simulink model "SGBMDisparityExample_original"  (R2021a)
settings: Solver=FixedStepDiscrete  StartTime=0.0  StopTime=simT  FixedStep=1  RelTol=1e-3
PreLoadFcn:
  | DL128 = Simulink.Variant('disparityLevels==128');
  | 
  | DLnot128 = Simulink.Variant('disparityLevels ~= 128');
  | 
  | disparityLevels = 64;
  | 
  | imgRowSize = 480;
  | 
  | imgColSize = 640;
  | 
  | P2 = 200; % Smoothness Penalty Large
  | P1 = 15;  % Smoothness Penalty Small
  | 
  | disparityFactor = 16;
  | 
  | uniquenessRatio = 5;
  | 
  | p = imgColSize - 1;
  | q = imgRowSize * imgColSize -1;
  | r = imgColSize - disparityLevels -1;
  | s = (imgRowSize*(imgColSize-disparityLevels))-1;
  | 
  | simT = 800*525
  | 
  | dtGain = 4;
InitFcn:
  | DL128 = Simulink.Variant('disparityLevels==128');
  | 
  | DLnot128 = Simulink.Variant('disparityLevels ~= 128');
  | 
  | img = imread(get_param('SGBMDisparityExample/leftImage','FileName'));
  | 
  | [imgRowSize, imgColSize] = size(img);
  | 
  | P2 = 200; % Smoothness Penalty Large
  | P1 = 15;  % Smoothness Penalty Small
  | 
  | disparityFactor = 16;
  | 
  | uniquenessRatio = str2num(get_param('SGBMDisparityExample/SGBMHDLAlgorithm','UT'));
  | 
  | disparityLevels = str2num(get_param('SGBMDisparityExample/SGBMHDLAlgorithm','DL'));
  | 
  | p = imgColSize - 1;
  | q = imgRowSize * imgColSize -1;
  | r = imgColSize - disparityLevels -1;
  | s = (imgRowSize*(imgColSize-disparityLevels))-1;
  | 
  | if imgRowSize == 720 && imgColSize == 1280
  | simT = 1650*750;
  | elseif imgRowSize == 540 && imgColSize == 960
  | simT = 1050*600;
  | elseif imgRowSize == 480 && imgColSize == 640
  | simT = 800*525;
  | end
  | 
  | if imgRowSize == 720 && imgColSize == 1280
  | dtGain = 2;
  | elseif imgRowSize == 540 && imgColSize == 960
  | dtGain = 2.6;
  | elseif imgRowSize == 480 && imgColSize == 640
  | dtGain = 4;
  | end
libraries: simulink x331, hdlsllib x105, visionhdlutilities x10, visionhdlio x4, visionsources x3
(part 6 of 6)

== system SGBMDisparityExample_original/SGBMHDLAlgorithm/PostProcessing/Interpolation/Division/QuoRem/Last ==
  In1 : Inport
  In2 : Inport  Port=2
  In3 : Inport  Port=3
  Add : Sum  OutDataTypeStr=fixdt(0,13,0)
  Add1 : Sum  Inputs=+-  OutDataTypeStr=fixdt(0,13,0)
  Add2 : Sum  OutDataTypeStr=fixdt(0,13,0)
  Bit Shift : hdlsllib/Logic and Bit Operations/Bit Shift  mode=Shift Left Logical  N=1
  Bitwise Operator : simulink/Logic and Bit Operations/Bitwise Operator  logicop=OR  UseBitMask=on  BitMask=bin2dec('0000')  BitMaskRealWorld=Stored Integer
  Bitwise Operator2 : simulink/Logic and Bit Operations/Bitwise Operator  logicop=OR  UseBitMask=on  BitMask=bin2dec('0001')  BitMaskRealWorld=Stored Integer
  Extract Bits{1..2,5..6} (4 alike) : simulink/Logic and Bit Operations/Extract Bits  bitsToExtract=Range starting with most significant bit  numBits=1  bitIdxRange=[7]  outScalingMode=Treat bit field as an integer
  Extract Bits3 : simulink/Logic and Bit Operations/Extract Bits  bitsToExtract=Upper half  numBits=8  bitIdxRange=[7]  outScalingMode=Treat bit field as an integer
  Extract Bits4 : simulink/Logic and Bit Operations/Extract Bits  bitsToExtract=Lower half  numBits=8  bitIdxRange=[7]  outScalingMode=Treat bit field as an integer
  Logical Operator : Logic  Operator=OR  AllPortsSameDT=off  OutDataTypeStr=boolean
  Switch{,1..4} (5 alike) : Switch  Criteria=u2 ~= 0
  Quo : Outport  VectorParamsAs1DForOutWhenUnconnected=off
  Div : Outport  Port=2  VectorParamsAs1DForOutWhenUnconnected=off
  Rem : Outport  Port=3  VectorParamsAs1DForOutWhenUnconnected=off
  wires:
  Add/1 -> Switch/1
  Bitwise Operator2/1 -> Switch1/3
  Bitwise Operator/1 -> Switch1/1
  Extract Bits2/1 -> Switch1/2
  Add1/1 -> Switch/3
  Extract Bits5/1 -> Switch2/2
  Add2/1 -> Switch2/1
  In1/1 -> Extract Bits1/1, Bit Shift/1
  Bit Shift/1 -> Extract Bits4/1, Extract Bits3/1
  Extract Bits3/1 -> Switch3/3, Add1/1, Add/1
  Extract Bits1/1 -> Switch/2
  Extract Bits4/1 -> Switch4/3, Extract Bits6/1, Bitwise Operator2/1, Bitwise Operator/1
  Switch/1 -> Extract Bits5/1, Add2/1, Extract Bits2/1, Switch2/3
  In2/1 -> Div/1, Add1/2, Add2/2, Add/2
  Switch3/1 -> Rem/1
  Switch4/1 -> Quo/1
  Extract Bits6/1 -> Logical Operator/1
  In3/1 -> Logical Operator/2
  Logical Operator/1 -> Switch3/2, Switch4/2
  Switch1/1 -> Switch4/1
  Switch2/1 -> Switch3/1

== system SGBMDisparityExample_original/SGBMHDLAlgorithm/PostProcessing/Interpolation/Division/QuoRem/Subsystem10 ==
  In1 : Inport
  In2 : Inport  Port=2
  In3 : Inport  Port=3
  Add : Sum  OutDataTypeStr=fixdt(0,13,0)
  Add1 : Sum  Inputs=+-  OutDataTypeStr=fixdt(0,13,0)
  Bit Concat2 : hdlsllib/Logic and Bit Operations/Bit Concat  numInputs=2
  Bit Shift : hdlsllib/Logic and Bit Operations/Bit Shift  mode=Shift Left Logical  N=1
  Bitwise Operator : simulink/Logic and Bit Operations/Bitwise Operator  logicop=OR  UseBitMask=on  BitMask=bin2dec('0')  BitMaskRealWorld=Stored Integer
  Bitwise Operator2 : simulink/Logic and Bit Operations/Bitwise Operator  logicop=OR  UseBitMask=on  BitMask=bin2dec('1')  BitMaskRealWorld=Stored Integer
  Extract Bits1 : simulink/Logic and Bit Operations/Extract Bits  bitsToExtract=Range starting with most significant bit  numBits=1  bitIdxRange=[7]  outScalingMode=Treat bit field as an integer
  Extract Bits2 : simulink/Logic and Bit Operations/Extract Bits  bitsToExtract=Range starting with most significant bit  numBits=1  bitIdxRange=[7]  outScalingMode=Treat bit field as an integer
  Extract Bits3 : simulink/Logic and Bit Operations/Extract Bits  bitsToExtract=Upper half  numBits=8  bitIdxRange=[7]  outScalingMode=Treat bit field as an integer
  Extract Bits4 : simulink/Logic and Bit Operations/Extract Bits  bitsToExtract=Lower half  numBits=8  bitIdxRange=[7]  outScalingMode=Treat bit field as an integer
  Extract Bits5 : simulink/Logic and Bit Operations/Extract Bits  bitsToExtract=Range starting with most significant bit  numBits=1  bitIdxRange=[7]  outScalingMode=Treat bit field as an integer
  Logical Operator : Logic  Operator=OR  AllPortsSameDT=off  OutDataTypeStr=boolean
  Switch : Switch  Criteria=u2 ~= 0
  Switch1 : Switch  Criteria=u2 ~= 0
  Switch2 : Switch  Criteria=u2 ~= 0
  Out1 : Outport  VectorParamsAs1DForOutWhenUnconnected=off
  Out2 : Outport  Port=2  VectorParamsAs1DForOutWhenUnconnected=off
  Start : Outport  Port=3  VectorParamsAs1DForOutWhenUnconnected=off
  wires:
  Add/1 -> Switch/1
  Bitwise Operator2/1 -> Switch1/3
  Bitwise Operator/1 -> Switch1/1
  Extract Bits2/1 -> Switch1/2
  Add1/1 -> Switch/3
  In1/1 -> Extract Bits1/1, Bit Shift/1
  Bit Shift/1 -> Extract Bits4/1, Extract Bits3/1, Switch2/3
  Extract Bits1/1 -> Switch/2
  Extract Bits3/1 -> Add1/1, Add/1
  Switch/1 -> Bit Concat2/1, Extract Bits2/1
  Switch1/1 -> Bit Concat2/2
  In2/1 -> Out2/1, Add1/2, Add/2
  Extract Bits4/1 -> Extract Bits5/1, Bitwise Operator2/1, Bitwise Operator/1
  Switch2/1 -> Out1/1
  Bit Concat2/1 -> Switch2/1
  Extract Bits5/1 -> Logical Operator/1
  In3/1 -> Logical Operator/2
  Logical Operator/1 -> Switch2/2, Start/1

== system SGBMDisparityExample_original/SGBMHDLAlgorithm/PostProcessing/Interpolation/Division/QuoRem/Subsystem11 ==
  In1 : Inport
  In2 : Inport  Port=2
  In3 : Inport  Port=3
  Add : Sum  OutDataTypeStr=fixdt(0,13,0)
  Add1 : Sum  Inputs=+-  OutDataTypeStr=fixdt(0,13,0)
  Bit Concat2 : hdlsllib/Logic and Bit Operations/Bit Concat  numInputs=2
  Bit Shift : hdlsllib/Logic and Bit Operations/Bit Shift  mode=Shift Left Logical  N=1
  Bitwise Operator : simulink/Logic and Bit Operations/Bitwise Operator  logicop=OR  UseBitMask=on  BitMask=bin2dec('0')  BitMaskRealWorld=Stored Integer
  Bitwise Operator2 : simulink/Logic and Bit Operations/Bitwise Operator  logicop=OR  UseBitMask=on  BitMask=bin2dec('1')  BitMaskRealWorld=Stored Integer
  Extract Bits1 : simulink/Logic and Bit Operations/Extract Bits  bitsToExtract=Range starting with most significant bit  numBits=1  bitIdxRange=[7]  outScalingMode=Treat bit field as an integer
  Extract Bits2 : simulink/Logic and Bit Operations/Extract Bits  bitsToExtract=Range starting with most significant bit  numBits=1  bitIdxRange=[7]  outScalingMode=Treat bit field as an integer
  Extract Bits3 : simulink/Logic and Bit Operations/Extract Bits  bitsToExtract=Upper half  numBits=8  bitIdxRange=[7]  outScalingMode=Treat bit field as an integer
  Extract Bits4 : simulink/Logic and Bit Operations/Extract Bits  bitsToExtract=Lower half  numBits=8  bitIdxRange=[7]  outScalingMode=Treat bit field as an integer
  Extract Bits5 : simulink/Logic and Bit Operations/Extract Bits  bitsToExtract=Range starting with most significant bit  numBits=1  bitIdxRange=[7]  outScalingMode=Treat bit field as an integer
  Logical Operator : Logic  Operator=OR  AllPortsSameDT=off  OutDataTypeStr=boolean
  Switch : Switch  Criteria=u2 ~= 0
  Switch1 : Switch  Criteria=u2 ~= 0
  Switch2 : Switch  Criteria=u2 ~= 0
  Out1 : Outport  VectorParamsAs1DForOutWhenUnconnected=off
  Out2 : Outport  Port=2  VectorParamsAs1DForOutWhenUnconnected=off
  Start : Outport  Port=3  VectorParamsAs1DForOutWhenUnconnected=off
  wires:
  Add/1 -> Switch/1
  Bitwise Operator2/1 -> Switch1/3
  Bitwise Operator/1 -> Switch1/1
  Extract Bits2/1 -> Switch1/2
  Add1/1 -> Switch/3
  In1/1 -> Extract Bits1/1, Bit Shift/1
  Bit Shift/1 -> Extract Bits4/1, Extract Bits3/1, Switch2/3
  Extract Bits1/1 -> Switch/2
  Extract Bits3/1 -> Add1/1, Add/1
  Switch/1 -> Bit Concat2/1, Extract Bits2/1
  Switch1/1 -> Bit Concat2/2
  In2/1 -> Out2/1, Add1/2, Add/2
  Extract Bits4/1 -> Extract Bits5/1, Bitwise Operator2/1, Bitwise Operator/1
  Switch2/1 -> Out1/1
  Bit Concat2/1 -> Switch2/1
  Extract Bits5/1 -> Logical Operator/1
  In3/1 -> Logical Operator/2
  Logical Operator/1 -> Switch2/2, Start/1

== system SGBMDisparityExample_original/SGBMHDLAlgorithm/PostProcessing/Interpolation/Division/QuoRem/Subsystem12 ==
  In1 : Inport
  In2 : Inport  Port=2
  In3 : Inport  Port=3
  Add : Sum  OutDataTypeStr=fixdt(0,13,0)
  Add1 : Sum  Inputs=+-  OutDataTypeStr=fixdt(0,13,0)
  Bit Concat2 : hdlsllib/Logic and Bit Operations/Bit Concat  numInputs=2
  Bit Shift : hdlsllib/Logic and Bit Operations/Bit Shift  mode=Shift Left Logical  N=1
  Bitwise Operator : simulink/Logic and Bit Operations/Bitwise Operator  logicop=OR  UseBitMask=on  BitMask=bin2dec('0')  BitMaskRealWorld=Stored Integer
  Bitwise Operator2 : simulink/Logic and Bit Operations/Bitwise Operator  logicop=OR  UseBitMask=on  BitMask=bin2dec('1')  BitMaskRealWorld=Stored Integer
  Extract Bits1 : simulink/Logic and Bit Operations/Extract Bits  bitsToExtract=Range starting with most significant bit  numBits=1  bitIdxRange=[7]  outScalingMode=Treat bit field as an integer
  Extract Bits2 : simulink/Logic and Bit Operations/Extract Bits  bitsToExtract=Range starting with most significant bit  numBits=1  bitIdxRange=[7]  outScalingMode=Treat bit field as an integer
  Extract Bits3 : simulink/Logic and Bit Operations/Extract Bits  bitsToExtract=Upper half  numBits=8  bitIdxRange=[7]  outScalingMode=Treat bit field as an integer
  Extract Bits4 : simulink/Logic and Bit Operations/Extract Bits  bitsToExtract=Lower half  numBits=8  bitIdxRange=[7]  outScalingMode=Treat bit field as an integer
  Extract Bits5 : simulink/Logic and Bit Operations/Extract Bits  bitsToExtract=Range starting with most significant bit  numBits=1  bitIdxRange=[7]  outScalingMode=Treat bit field as an integer
  Logical Operator : Logic  Operator=OR  AllPortsSameDT=off  OutDataTypeStr=boolean
  Switch : Switch  Criteria=u2 ~= 0
  Switch1 : Switch  Criteria=u2 ~= 0
  Switch2 : Switch  Criteria=u2 ~= 0
  Out1 : Outport  VectorParamsAs1DForOutWhenUnconnected=off
  Out2 : Outport  Port=2  VectorParamsAs1DForOutWhenUnconnected=off
  Start : Outport  Port=3  VectorParamsAs1DForOutWhenUnconnected=off
  wires:
  Add/1 -> Switch/1
  Bitwise Operator2/1 -> Switch1/3
  Bitwise Operator/1 -> Switch1/1
  Extract Bits2/1 -> Switch1/2
  Add1/1 -> Switch/3
  In1/1 -> Extract Bits1/1, Bit Shift/1
  Bit Shift/1 -> Extract Bits4/1, Extract Bits3/1, Switch2/3
  Extract Bits1/1 -> Switch/2
  Extract Bits3/1 -> Add1/1, Add/1
  Switch/1 -> Bit Concat2/1, Extract Bits2/1
  Switch1/1 -> Bit Concat2/2
  In2/1 -> Out2/1, Add1/2, Add/2
  Extract Bits4/1 -> Extract Bits5/1, Bitwise Operator2/1, Bitwise Operator/1
  Switch2/1 -> Out1/1
  Bit Concat2/1 -> Switch2/1
  Extract Bits5/1 -> Logical Operator/1
  In3/1 -> Logical Operator/2
  Logical Operator/1 -> Switch2/2, Start/1

== system SGBMDisparityExample_original/SGBMHDLAlgorithm/PostProcessing/Interpolation/Division/QuoRem/Subsystem2 ==
  In1 : Inport
  In2 : Inport  Port=2
  In3 : Inport  Port=3
  Add : Sum  OutDataTypeStr=fixdt(0,13,0)
  Add1 : Sum  Inputs=+-  OutDataTypeStr=fixdt(0,13,0)
  Bit Concat2 : hdlsllib/Logic and Bit Operations/Bit Concat  numInputs=2
  Bit Shift : hdlsllib/Logic and Bit Operations/Bit Shift  mode=Shift Left Logical  N=1
  Bitwise Operator : simulink/Logic and Bit Operations/Bitwise Operator  logicop=OR  UseBitMask=on  BitMask=bin2dec('0')  BitMaskRealWorld=Stored Integer
  Bitwise Operator2 : simulink/Logic and Bit Operations/Bitwise Operator  logicop=OR  UseBitMask=on  BitMask=bin2dec('1')  BitMaskRealWorld=Stored Integer
  Extract Bits1 : simulink/Logic and Bit Operations/Extract Bits  bitsToExtract=Range starting with most significant bit  numBits=1  bitIdxRange=[7]  outScalingMode=Treat bit field as an integer
  Extract Bits2 : simulink/Logic and Bit Operations/Extract Bits  bitsToExtract=Range starting with most significant bit  numBits=1  bitIdxRange=[7]  outScalingMode=Treat bit field as an integer
  Extract Bits3 : simulink/Logic and Bit Operations/Extract Bits  bitsToExtract=Upper half  numBits=8  bitIdxRange=[7]  outScalingMode=Treat bit field as an integer
  Extract Bits4 : simulink/Logic and Bit Operations/Extract Bits  bitsToExtract=Lower half  numBits=8  bitIdxRange=[7]  outScalingMode=Treat bit field as an integer
  Extract Bits5 : simulink/Logic and Bit Operations/Extract Bits  bitsToExtract=Range starting with most significant bit  numBits=1  bitIdxRange=[7]  outScalingMode=Treat bit field as an integer
  Logical Operator : Logic  Operator=OR  AllPortsSameDT=off  OutDataTypeStr=boolean
  Switch : Switch  Criteria=u2 ~= 0
  Switch1 : Switch  Criteria=u2 ~= 0
  Switch2 : Switch  Criteria=u2 ~= 0
  Out1 : Outport  VectorParamsAs1DForOutWhenUnconnected=off
  Out2 : Outport  Port=2  VectorParamsAs1DForOutWhenUnconnected=off
  Start : Outport  Port=3  VectorParamsAs1DForOutWhenUnconnected=off
  wires:
  Add/1 -> Switch/1
  Bitwise Operator2/1 -> Switch1/3
  Bitwise Operator/1 -> Switch1/1
  Extract Bits2/1 -> Switch1/2
  Add1/1 -> Switch/3
  In1/1 -> Extract Bits1/1, Bit Shift/1
  Bit Shift/1 -> Extract Bits4/1, Extract Bits3/1, Switch2/3
  Extract Bits1/1 -> Switch/2
  Extract Bits3/1 -> Add1/1, Add/1
  Switch/1 -> Bit Concat2/1, Extract Bits2/1
  Switch1/1 -> Bit Concat2/2
  In2/1 -> Out2/1, Add1/2, Add/2
  Extract Bits4/1 -> Extract Bits5/1, Bitwise Operator2/1, Bitwise Operator/1
  Switch2/1 -> Out1/1
  Bit Concat2/1 -> Switch2/1
  Extract Bits5/1 -> Logical Operator/1
  In3/1 -> Logical Operator/2
  Logical Operator/1 -> Switch2/2, Start/1

== system SGBMDisparityExample_original/SGBMHDLAlgorithm/PostProcessing/Interpolation/Division/QuoRem/Subsystem3 ==
  In1 : Inport
  In2 : Inport  Port=2
  In3 : Inport  Port=3
  Add : Sum  OutDataTypeStr=fixdt(0,13,0)
  Add1 : Sum  Inputs=+-  OutDataTypeStr=fixdt(0,13,0)
  Bit Concat2 : hdlsllib/Logic and Bit Operations/Bit Concat  numInputs=2
  Bit Shift : hdlsllib/Logic and Bit Operations/Bit Shift  mode=Shift Left Logical  N=1
  Bitwise Operator : simulink/Logic and Bit Operations/Bitwise Operator  logicop=OR  UseBitMask=on  BitMask=bin2dec('0')  BitMaskRealWorld=Stored Integer
  Bitwise Operator2 : simulink/Logic and Bit Operations/Bitwise Operator  logicop=OR  UseBitMask=on  BitMask=bin2dec('1')  BitMaskRealWorld=Stored Integer
  Extract Bits1 : simulink/Logic and Bit Operations/Extract Bits  bitsToExtract=Range starting with most significant bit  numBits=1  bitIdxRange=[7]  outScalingMode=Treat bit field as an integer
  Extract Bits2 : simulink/Logic and Bit Operations/Extract Bits  bitsToExtract=Range starting with most significant bit  numBits=1  bitIdxRange=[7]  outScalingMode=Treat bit field as an integer
  Extract Bits3 : simulink/Logic and Bit Operations/Extract Bits  bitsToExtract=Upper half  numBits=8  bitIdxRange=[7]  outScalingMode=Treat bit field as an integer
  Extract Bits4 : simulink/Logic and Bit Operations/Extract Bits  bitsToExtract=Lower half  numBits=8  bitIdxRange=[7]  outScalingMode=Treat bit field as an integer
  Extract Bits5 : simulink/Logic and Bit Operations/Extract Bits  bitsToExtract=Range starting with most significant bit  numBits=1  bitIdxRange=[7]  outScalingMode=Treat bit field as an integer
  Logical Operator : Logic  Operator=OR  AllPortsSameDT=off  OutDataTypeStr=boolean
  Switch : Switch  Criteria=u2 ~= 0
  Switch1 : Switch  Criteria=u2 ~= 0
  Switch2 : Switch  Criteria=u2 ~= 0
  Out1 : Outport  VectorParamsAs1DForOutWhenUnconnected=off
  Out2 : Outport  Port=2  VectorParamsAs1DForOutWhenUnconnected=off
  Start : Outport  Port=3  VectorParamsAs1DForOutWhenUnconnected=off
  wires:
  Add/1 -> Switch/1
  Bitwise Operator2/1 -> Switch1/3
  Bitwise Operator/1 -> Switch1/1
  Extract Bits2/1 -> Switch1/2
  Add1/1 -> Switch/3
  In1/1 -> Extract Bits1/1, Bit Shift/1
  Bit Shift/1 -> Extract Bits4/1, Extract Bits3/1, Switch2/3
  Extract Bits1/1 -> Switch/2
  Extract Bits3/1 -> Add1/1, Add/1
  Switch/1 -> Bit Concat2/1, Extract Bits2/1
  Switch1/1 -> Bit Concat2/2
  In2/1 -> Out2/1, Add1/2, Add/2
  Extract Bits4/1 -> Extract Bits5/1, Bitwise Operator2/1, Bitwise Operator/1
  Switch2/1 -> Out1/1
  Bit Concat2/1 -> Switch2/1
  Extract Bits5/1 -> Logical Operator/1
  In3/1 -> Logical Operator/2
  Logical Operator/1 -> Switch2/2, Start/1

== system SGBMDisparityExample_original/SGBMHDLAlgorithm/PostProcessing/Interpolation/Division/QuoRem/Subsystem4 ==
  In1 : Inport
  In2 : Inport  Port=2
  In3 : Inport  Port=3
  Add : Sum  OutDataTypeStr=fixdt(0,13,0)
  Add1 : Sum  Inputs=+-  OutDataTypeStr=fixdt(0,13,0)
  Bit Concat2 : hdlsllib/Logic and Bit Operations/Bit Concat  numInputs=2
  Bit Shift : hdlsllib/Logic and Bit Operations/Bit Shift  mode=Shift Left Logical  N=1
  Bitwise Operator : simulink/Logic and Bit Operations/Bitwise Operator  logicop=OR  UseBitMask=on  BitMask=bin2dec('0')  BitMaskRealWorld=Stored Integer
  Bitwise Operator2 : simulink/Logic and Bit Operations/Bitwise Operator  logicop=OR  UseBitMask=on  BitMask=bin2dec('1')  BitMaskRealWorld=Stored Integer
  Extract Bits1 : simulink/Logic and Bit Operations/Extract Bits  bitsToExtract=Range starting with most significant bit  numBits=1  bitIdxRange=[7]  outScalingMode=Treat bit field as an integer
  Extract Bits2 : simulink/Logic and Bit Operations/Extract Bits  bitsToExtract=Range starting with most significant bit  numBits=1  bitIdxRange=[7]  outScalingMode=Treat bit field as an integer
  Extract Bits3 : simulink/Logic and Bit Operations/Extract Bits  bitsToExtract=Upper half  numBits=8  bitIdxRange=[7]  outScalingMode=Treat bit field as an integer
  Extract Bits4 : simulink/Logic and Bit Operations/Extract Bits  bitsToExtract=Lower half  numBits=8  bitIdxRange=[7]  outScalingMode=Treat bit field as an integer
  Extract Bits5 : simulink/Logic and Bit Operations/Extract Bits  bitsToExtract=Range starting with most significant bit  numBits=1  bitIdxRange=[7]  outScalingMode=Treat bit field as an integer
  Logical Operator : Logic  Operator=OR  AllPortsSameDT=off  OutDataTypeStr=boolean
  Switch : Switch  Criteria=u2 ~= 0
  Switch1 : Switch  Criteria=u2 ~= 0
  Switch2 : Switch  Criteria=u2 ~= 0
  Out1 : Outport  VectorParamsAs1DForOutWhenUnconnected=off
  Out2 : Outport  Port=2  VectorParamsAs1DForOutWhenUnconnected=off
  Start : Outport  Port=3  VectorParamsAs1DForOutWhenUnconnected=off
  wires:
  Add/1 -> Switch/1
  Bitwise Operator2/1 -> Switch1/3
  Bitwise Operator/1 -> Switch1/1
  Extract Bits2/1 -> Switch1/2
  Add1/1 -> Switch/3
  In1/1 -> Extract Bits1/1, Bit Shift/1
  Bit Shift/1 -> Extract Bits4/1, Extract Bits3/1, Switch2/3
  Extract Bits1/1 -> Switch/2
  Extract Bits3/1 -> Add1/1, Add/1
  Switch/1 -> Bit Concat2/1, Extract Bits2/1
  Switch1/1 -> Bit Concat2/2
  In2/1 -> Out2/1, Add1/2, Add/2
  Extract Bits4/1 -> Extract Bits5/1, Bitwise Operator2/1, Bitwise Operator/1
  Switch2/1 -> Out1/1
  Bit Concat2/1 -> Switch2/1
  Extract Bits5/1 -> Logical Operator/1
  In3/1 -> Logical Operator/2
  Logical Operator/1 -> Switch2/2, Start/1

== system SGBMDisparityExample_original/SGBMHDLAlgorithm/PostProcessing/Interpolation/Division/QuoRem/Subsystem5 ==
  In1 : Inport
  In2 : Inport  Port=2
  In3 : Inport  Port=3
  Add : Sum  OutDataTypeStr=fixdt(0,13,0)
  Add1 : Sum  Inputs=+-  OutDataTypeStr=fixdt(0,13,0)
  Bit Concat2 : hdlsllib/Logic and Bit Operations/Bit Concat  numInputs=2
  Bit Shift : hdlsllib/Logic and Bit Operations/Bit Shift  mode=Shift Left Logical  N=1
  Bitwise Operator : simulink/Logic and Bit Operations/Bitwise Operator  logicop=OR  UseBitMask=on  BitMask=bin2dec('0')  BitMaskRealWorld=Stored Integer
  Bitwise Operator2 : simulink/Logic and Bit Operations/Bitwise Operator  logicop=OR  UseBitMask=on  BitMask=bin2dec('1')  BitMaskRealWorld=Stored Integer
  Extract Bits1 : simulink/Logic and Bit Operations/Extract Bits  bitsToExtract=Range starting with most significant bit  numBits=1  bitIdxRange=[7]  outScalingMode=Treat bit field as an integer
  Extract Bits2 : simulink/Logic and Bit Operations/Extract Bits  bitsToExtract=Range starting with most significant bit  numBits=1  bitIdxRange=[7]  outScalingMode=Treat bit field as an integer
  Extract Bits3 : simulink/Logic and Bit Operations/Extract Bits  bitsToExtract=Upper half  numBits=8  bitIdxRange=[7]  outScalingMode=Treat bit field as an integer
  Extract Bits4 : simulink/Logic and Bit Operations/Extract Bits  bitsToExtract=Lower half  numBits=8  bitIdxRange=[7]  outScalingMode=Treat bit field as an integer
  Extract Bits5 : simulink/Logic and Bit Operations/Extract Bits  bitsToExtract=Range starting with most significant bit  numBits=1  bitIdxRange=[7]  outScalingMode=Treat bit field as an integer
  Logical Operator : Logic  Operator=OR  AllPortsSameDT=off  OutDataTypeStr=boolean
  Switch : Switch  Criteria=u2 ~= 0
  Switch1 : Switch  Criteria=u2 ~= 0
  Switch2 : Switch  Criteria=u2 ~= 0
  Out1 : Outport  VectorParamsAs1DForOutWhenUnconnected=off
  Out2 : Outport  Port=2  VectorParamsAs1DForOutWhenUnconnected=off
  Start : Outport  Port=3  VectorParamsAs1DForOutWhenUnconnected=off
  wires:
  Add/1 -> Switch/1
  Bitwise Operator2/1 -> Switch1/3
  Bitwise Operator/1 -> Switch1/1
  Extract Bits2/1 -> Switch1/2
  Add1/1 -> Switch/3
  In1/1 -> Extract Bits1/1, Bit Shift/1
  Bit Shift/1 -> Extract Bits4/1, Extract Bits3/1, Switch2/3
  Extract Bits1/1 -> Switch/2
  Extract Bits3/1 -> Add1/1, Add/1
  Switch/1 -> Bit Concat2/1, Extract Bits2/1
  Switch1/1 -> Bit Concat2/2
  In2/1 -> Out2/1, Add1/2, Add/2
  Extract Bits4/1 -> Extract Bits5/1, Bitwise Operator2/1, Bitwise Operator/1
  Switch2/1 -> Out1/1
  Bit Concat2/1 -> Switch2/1
  Extract Bits5/1 -> Logical Operator/1
  In3/1 -> Logical Operator/2
  Logical Operator/1 -> Switch2/2, Start/1

== system SGBMDisparityExample_original/SGBMHDLAlgorithm/PostProcessing/Interpolation/Division/QuoRem/Subsystem6 ==
  In1 : Inport
  In2 : Inport  Port=2
  In3 : Inport  Port=3
  Add : Sum  OutDataTypeStr=fixdt(0,13,0)
  Add1 : Sum  Inputs=+-  OutDataTypeStr=fixdt(0,13,0)
  Bit Concat2 : hdlsllib/Logic and Bit Operations/Bit Concat  numInputs=2
  Bit Shift : hdlsllib/Logic and Bit Operations/Bit Shift  mode=Shift Left Logical  N=1
  Bitwise Operator : simulink/Logic and Bit Operations/Bitwise Operator  logicop=OR  UseBitMask=on  BitMask=bin2dec('0')  BitMaskRealWorld=Stored Integer
  Bitwise Operator2 : simulink/Logic and Bit Operations/Bitwise Operator  logicop=OR  UseBitMask=on  BitMask=bin2dec('1')  BitMaskRealWorld=Stored Integer
  Extract Bits1 : simulink/Logic and Bit Operations/Extract Bits  bitsToExtract=Range starting with most significant bit  numBits=1  bitIdxRange=[7]  outScalingMode=Treat bit field as an integer
  Extract Bits2 : simulink/Logic and Bit Operations/Extract Bits  bitsToExtract=Range starting with most significant bit  numBits=1  bitIdxRange=[7]  outScalingMode=Treat bit field as an integer
  Extract Bits3 : simulink/Logic and Bit Operations/Extract Bits  bitsToExtract=Upper half  numBits=8  bitIdxRange=[7]  outScalingMode=Treat bit field as an integer
  Extract Bits4 : simulink/Logic and Bit Operations/Extract Bits  bitsToExtract=Lower half  numBits=8  bitIdxRange=[7]  outScalingMode=Treat bit field as an integer
  Extract Bits5 : simulink/Logic and Bit Operations/Extract Bits  bitsToExtract=Range starting with most significant bit  numBits=1  bitIdxRange=[7]  outScalingMode=Treat bit field as an integer
  Logical Operator : Logic  Operator=OR  AllPortsSameDT=off  OutDataTypeStr=boolean
  Switch : Switch  Criteria=u2 ~= 0
  Switch1 : Switch  Criteria=u2 ~= 0
  Switch2 : Switch  Criteria=u2 ~= 0
  Out1 : Outport  VectorParamsAs1DForOutWhenUnconnected=off
  Out2 : Outport  Port=2  VectorParamsAs1DForOutWhenUnconnected=off
  Start : Outport  Port=3  VectorParamsAs1DForOutWhenUnconnected=off
  wires:
  Add/1 -> Switch/1
  Bitwise Operator2/1 -> Switch1/3
  Bitwise Operator/1 -> Switch1/1
  Extract Bits2/1 -> Switch1/2
  Add1/1 -> Switch/3
  In1/1 -> Extract Bits1/1, Bit Shift/1
  Bit Shift/1 -> Extract Bits4/1, Extract Bits3/1, Switch2/3
  Extract Bits1/1 -> Switch/2
  Extract Bits3/1 -> Add1/1, Add/1
  Switch/1 -> Bit Concat2/1, Extract Bits2/1
  Switch1/1 -> Bit Concat2/2
  In2/1 -> Out2/1, Add1/2, Add/2
  Extract Bits4/1 -> Extract Bits5/1, Bitwise Operator2/1, Bitwise Operator/1
  Switch2/1 -> Out1/1
  Bit Concat2/1 -> Switch2/1
  Extract Bits5/1 -> Logical Operator/1
  In3/1 -> Logical Operator/2
  Logical Operator/1 -> Switch2/2, Start/1

== system SGBMDisparityExample_original/SGBMHDLAlgorithm/PostProcessing/Interpolation/Division/QuoRem/Subsystem7 ==
  In1 : Inport
  In2 : Inport  Port=2
  In3 : Inport  Port=3
  Add : Sum  OutDataTypeStr=fixdt(0,13,0)
  Add1 : Sum  Inputs=+-  OutDataTypeStr=fixdt(0,13,0)
  Bit Concat2 : hdlsllib/Logic and Bit Operations/Bit Concat  numInputs=2
  Bit Shift : hdlsllib/Logic and Bit Operations/Bit Shift  mode=Shift Left Logical  N=1
  Bitwise Operator : simulink/Logic and Bit Operations/Bitwise Operator  logicop=OR  UseBitMask=on  BitMask=bin2dec('0')  BitMaskRealWorld=Stored Integer
  Bitwise Operator2 : simulink/Logic and Bit Operations/Bitwise Operator  logicop=OR  UseBitMask=on  BitMask=bin2dec('1')  BitMaskRealWorld=Stored Integer
  Extract Bits1 : simulink/Logic and Bit Operations/Extract Bits  bitsToExtract=Range starting with most significant bit  numBits=1  bitIdxRange=[7]  outScalingMode=Treat bit field as an integer
  Extract Bits2 : simulink/Logic and Bit Operations/Extract Bits  bitsToExtract=Range starting with most significant bit  numBits=1  bitIdxRange=[7]  outScalingMode=Treat bit field as an integer
  Extract Bits3 : simulink/Logic and Bit Operations/Extract Bits  bitsToExtract=Upper half  numBits=8  bitIdxRange=[7]  outScalingMode=Treat bit field as an integer
  Extract Bits4 : simulink/Logic and Bit Operations/Extract Bits  bitsToExtract=Lower half  numBits=8  bitIdxRange=[7]  outScalingMode=Treat bit field as an integer
  Extract Bits5 : simulink/Logic and Bit Operations/Extract Bits  bitsToExtract=Range starting with most significant bit  numBits=1  bitIdxRange=[7]  outScalingMode=Treat bit field as an integer
  Logical Operator : Logic  Operator=OR  AllPortsSameDT=off  OutDataTypeStr=boolean
  Switch : Switch  Criteria=u2 ~= 0
  Switch1 : Switch  Criteria=u2 ~= 0
  Switch2 : Switch  Criteria=u2 ~= 0
  Out1 : Outport  VectorParamsAs1DForOutWhenUnconnected=off
  Out2 : Outport  Port=2  VectorParamsAs1DForOutWhenUnconnected=off
  Start : Outport  Port=3  VectorParamsAs1DForOutWhenUnconnected=off
  wires:
  Add/1 -> Switch/1
  Bitwise Operator2/1 -> Switch1/3
  Bitwise Operator/1 -> Switch1/1
  Extract Bits2/1 -> Switch1/2
  Add1/1 -> Switch/3
  In1/1 -> Extract Bits1/1, Bit Shift/1
  Bit Shift/1 -> Extract Bits4/1, Extract Bits3/1, Switch2/3
  Extract Bits1/1 -> Switch/2
  Extract Bits3/1 -> Add1/1, Add/1
  Switch/1 -> Bit Concat2/1, Extract Bits2/1
  Switch1/1 -> Bit Concat2/2
  In2/1 -> Out2/1, Add1/2, Add/2
  Extract Bits4/1 -> Extract Bits5/1, Bitwise Operator2/1, Bitwise Operator/1
  Switch2/1 -> Out1/1
  Bit Concat2/1 -> Switch2/1
  Extract Bits5/1 -> Logical Operator/1
  In3/1 -> Logical Operator/2
  Logical Operator/1 -> Switch2/2, Start/1

== system SGBMDisparityExample_original/SGBMHDLAlgorithm/PostProcessing/Interpolation/Division/QuoRem/Subsystem8 ==
  In1 : Inport
  In2 : Inport  Port=2
  In3 : Inport  Port=3
  Add : Sum  OutDataTypeStr=fixdt(0,13,0)
  Add1 : Sum  Inputs=+-  OutDataTypeStr=fixdt(0,13,0)
  Bit Concat2 : hdlsllib/Logic and Bit Operations/Bit Concat  numInputs=2
  Bit Shift : hdlsllib/Logic and Bit Operations/Bit Shift  mode=Shift Left Logical  N=1
  Bitwise Operator : simulink/Logic and Bit Operations/Bitwise Operator  logicop=OR  UseBitMask=on  BitMask=bin2dec('0')  BitMaskRealWorld=Stored Integer
  Bitwise Operator2 : simulink/Logic and Bit Operations/Bitwise Operator  logicop=OR  UseBitMask=on  BitMask=bin2dec('1')  BitMaskRealWorld=Stored Integer
  Extract Bits1 : simulink/Logic and Bit Operations/Extract Bits  bitsToExtract=Range starting with most significant bit  numBits=1  bitIdxRange=[7]  outScalingMode=Treat bit field as an integer
  Extract Bits2 : simulink/Logic and Bit Operations/Extract Bits  bitsToExtract=Range starting with most significant bit  numBits=1  bitIdxRange=[7]  outScalingMode=Treat bit field as an integer
  Extract Bits3 : simulink/Logic and Bit Operations/Extract Bits  bitsToExtract=Upper half  numBits=8  bitIdxRange=[7]  outScalingMode=Treat bit field as an integer
  Extract Bits4 : simulink/Logic and Bit Operations/Extract Bits  bitsToExtract=Lower half  numBits=8  bitIdxRange=[7]  outScalingMode=Treat bit field as an integer
  Extract Bits5 : simulink/Logic and Bit Operations/Extract Bits  bitsToExtract=Range starting with most significant bit  numBits=1  bitIdxRange=[7]  outScalingMode=Treat bit field as an integer
  Logical Operator : Logic  Operator=OR  AllPortsSameDT=off  OutDataTypeStr=boolean
  Switch : Switch  Criteria=u2 ~= 0
  Switch1 : Switch  Criteria=u2 ~= 0
  Switch2 : Switch  Criteria=u2 ~= 0
  Out1 : Outport  VectorParamsAs1DForOutWhenUnconnected=off
  Out2 : Outport  Port=2  VectorParamsAs1DForOutWhenUnconnected=off
  Start : Outport  Port=3  VectorParamsAs1DForOutWhenUnconnected=off
  wires:
  Add/1 -> Switch/1
  Bitwise Operator2/1 -> Switch1/3
  Bitwise Operator/1 -> Switch1/1
  Extract Bits2/1 -> Switch1/2
  Add1/1 -> Switch/3
  In1/1 -> Extract Bits1/1, Bit Shift/1
  Bit Shift/1 -> Extract Bits4/1, Extract Bits3/1, Switch2/3
  Extract Bits1/1 -> Switch/2
  Extract Bits3/1 -> Add1/1, Add/1
  Switch/1 -> Bit Concat2/1, Extract Bits2/1
  Switch1/1 -> Bit Concat2/2
  In2/1 -> Out2/1, Add1/2, Add/2
  Extract Bits4/1 -> Extract Bits5/1, Bitwise Operator2/1, Bitwise Operator/1
  Switch2/1 -> Out1/1
  Bit Concat2/1 -> Switch2/1
  Extract Bits5/1 -> Logical Operator/1
  In3/1 -> Logical Operator/2
  Logical Operator/1 -> Switch2/2, Start/1

== system SGBMDisparityExample_original/SGBMHDLAlgorithm/PostProcessing/Interpolation/Division/QuoRem/Subsystem9 ==
  In1 : Inport
  In2 : Inport  Port=2
  In3 : Inport  Port=3
  Add : Sum  OutDataTypeStr=fixdt(0,13,0)
  Add1 : Sum  Inputs=+-  OutDataTypeStr=fixdt(0,13,0)
  Bit Concat2 : hdlsllib/Logic and Bit Operations/Bit Concat  numInputs=2
  Bit Shift : hdlsllib/Logic and Bit Operations/Bit Shift  mode=Shift Left Logical  N=1
  Bitwise Operator : simulink/Logic and Bit Operations/Bitwise Operator  logicop=OR  UseBitMask=on  BitMask=bin2dec('0')  BitMaskRealWorld=Stored Integer
  Bitwise Operator2 : simulink/Logic and Bit Operations/Bitwise Operator  logicop=OR  UseBitMask=on  BitMask=bin2dec('1')  BitMaskRealWorld=Stored Integer
  Extract Bits1 : simulink/Logic and Bit Operations/Extract Bits  bitsToExtract=Range starting with most significant bit  numBits=1  bitIdxRange=[7]  outScalingMode=Treat bit field as an integer
  Extract Bits2 : simulink/Logic and Bit Operations/Extract Bits  bitsToExtract=Range starting with most significant bit  numBits=1  bitIdxRange=[7]  outScalingMode=Treat bit field as an integer
  Extract Bits3 : simulink/Logic and Bit Operations/Extract Bits  bitsToExtract=Upper half  numBits=8  bitIdxRange=[7]  outScalingMode=Treat bit field as an integer
  Extract Bits4 : simulink/Logic and Bit Operations/Extract Bits  bitsToExtract=Lower half  numBits=8  bitIdxRange=[7]  outScalingMode=Treat bit field as an integer
  Extract Bits5 : simulink/Logic and Bit Operations/Extract Bits  bitsToExtract=Range starting with most significant bit  numBits=1  bitIdxRange=[7]  outScalingMode=Treat bit field as an integer
  Logical Operator : Logic  Operator=OR  AllPortsSameDT=off  OutDataTypeStr=boolean
  Switch : Switch  Criteria=u2 ~= 0
  Switch1 : Switch  Criteria=u2 ~= 0
  Switch2 : Switch  Criteria=u2 ~= 0
  Out1 : Outport  VectorParamsAs1DForOutWhenUnconnected=off
  Out2 : Outport  Port=2  VectorParamsAs1DForOutWhenUnconnected=off
  Start : Outport  Port=3  VectorParamsAs1DForOutWhenUnconnected=off
  wires:
  Add/1 -> Switch/1
  Bitwise Operator2/1 -> Switch1/3
  Bitwise Operator/1 -> Switch1/1
  Extract Bits2/1 -> Switch1/2
  Add1/1 -> Switch/3
  In1/1 -> Extract Bits1/1, Bit Shift/1
  Bit Shift/1 -> Extract Bits4/1, Extract Bits3/1, Switch2/3
  Extract Bits1/1 -> Switch/2
  Extract Bits3/1 -> Add1/1, Add/1
  Switch/1 -> Bit Concat2/1, Extract Bits2/1
  Switch1/1 -> Bit Concat2/2
  In2/1 -> Out2/1, Add1/2, Add/2
  Extract Bits4/1 -> Extract Bits5/1, Bitwise Operator2/1, Bitwise Operator/1
  Switch2/1 -> Out1/1
  Bit Concat2/1 -> Switch2/1
  Extract Bits5/1 -> Logical Operator/1
  In3/1 -> Logical Operator/2
  Logical Operator/1 -> Switch2/2, Start/1

== system SGBMDisparityExample_original/SGBMHDLAlgorithm/PostProcessing/Interpolation/Minimum_Cost_Index/DL_Vector/DL128 ==
  In1 : Inport
  Out1 : Outport  VectorParamsAs1DForOutWhenUnconnected=off
  wires:
  In1/1 -> Out1/1

== system SGBMDisparityExample_original/SGBMHDLAlgorithm/PostProcessing/Interpolation/Minimum_Cost_Index/DL_Vector/DLnot128 ==
  In1 : Inport
  Constants : Subsystem
  Mux27 : Mux  Inputs=2
  Selector50 : Selector  InputPortWidth=disparityLevels  IndexOptions=Index vector (dialog)  Indices=[1:disparityLevels]  OutputSizes=1
  Selector51 : Selector  InputPortWidth=128  IndexOptions=Index vector (dialog)  Indices=[disparityLevels+1:128]  OutputSizes=1
  Out1 : Outport  VectorParamsAs1DForOutWhenUnconnected=off
  wires:
  Mux27/1 -> Out1/1
  Constants/1(Out1) -> Selector51/1
  Selector51/1 -> Mux27/2
  In1/1 -> Selector50/1
  Selector50/1 -> Mux27/1

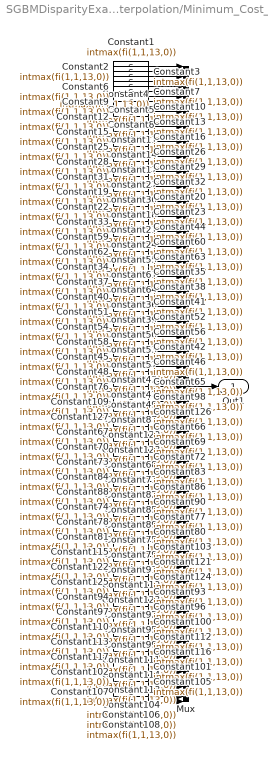
== system SGBMDisparityExample_original/SGBMHDLAlgorithm/PostProcessing/Interpolation/Minimum_Cost_Index/DL_Vector/DLnot128/Constants ==
  Constant{1..128} (128 alike) : Constant  Value=intmax(fi(1,1,13,0))  OutDataTypeStr=fixdt(1,13,0)  SampleTime=-1
  Mux : Mux  Inputs=128
  Out1 : Outport  VectorParamsAs1DForOutWhenUnconnected=off
  wires:
  Constant1/1 -> Mux/1
  Constant2/1 -> Mux/2
  Constant3/1 -> Mux/3
  Constant4/1 -> Mux/4
  Constant8/1 -> Mux/8
  Constant7/1 -> Mux/7
  Constant5/1 -> Mux/5
  Constant6/1 -> Mux/6
  Constant15/1 -> Mux/15
  Constant13/1 -> Mux/13
  Constant14/1 -> Mux/14
  Constant12/1 -> Mux/12
  Constant11/1 -> Mux/11
  Constant16/1 -> Mux/16
  Constant9/1 -> Mux/9
  Constant10/1 -> Mux/10
  Constant19/1 -> Mux/27
  Constant30/1 -> Mux/23
  Constant28/1 -> Mux/21
  Constant31/1 -> Mux/24
  Constant29/1 -> Mux/22
  Constant21/1 -> Mux/29
  Constant26/1 -> Mux/19
  Constant17/1 -> Mux/17
  Constant23/1 -> Mux/31
  Constant25/1 -> Mux/18
  Constant22/1 -> Mux/30
  Constant18/1 -> Mux/26
  Constant32/1 -> Mux/25
  Constant20/1 -> Mux/28
  Constant27/1 -> Mux/20
  Constant24/1 -> Mux/32
  Constant42/1 -> Mux/58
  Constant51/1 -> Mux/51
  Constant47/1 -> Mux/62
  Constant35/1 -> Mux/43
  Constant41/1 -> Mux/49
  Constant62/1 -> Mux/39
  Constant60/1 -> Mux/37
  Constant45/1 -> Mux/60
  Constant61/1 -> Mux/38
  Constant55/1 -> Mux/35
  Constant36/1 -> Mux/44
  Constant49/1 -> Mux/64
  Constant50/1 -> Mux/50
  Constant48/1 -> Mux/63
  Constant43/1 -> Mux/59
  Constant63/1 -> Mux/40
  Constant33/1 -> Mux/33
  Constant39/1 -> Mux/47
  Constant34/1 -> Mux/42
  Constant44/1 -> Mux/34
  Constant38/1 -> Mux/46
  Constant58/1 -> Mux/57
  Constant56/1 -> Mux/55
  Constant37/1 -> Mux/45
  Constant54/1 -> Mux/54
  Constant53/1 -> Mux/53
  Constant40/1 -> Mux/48
  Constant59/1 -> Mux/36
  Constant64/1 -> Mux/41
  Constant46/1 -> Mux/61
  Constant57/1 -> Mux/56
  Constant52/1 -> Mux/52
  Constant74/1 -> Mux/90
  Constant67/1 -> Mux/75
  Constant73/1 -> Mux/81
  Constant126/1 -> Mux/71
  Constant109/1 -> Mux/69
  Constant77/1 -> Mux/92
  Constant120/1 -> Mux/70
  Constant68/1 -> Mux/76
  Constant81/1 -> Mux/96
  Constant82/1 -> Mux/82
  Constant80/1 -> Mux/95
  Constant65/1 -> Mux/65
  Constant71/1 -> Mux/79
  Constant72/1 -> Mux/80
  Constant98/1 -> Mux/68
  Constant123/1 -> Mux/103
  Constant88/1 -> Mux/87
  Constant69/1 -> Mux/77
  Constant119/1 -> Mux/100
  Constant85/1 -> Mux/85
  Constant89/1 -> Mux/88
  Constant84/1 -> Mux/84
  Constant107/1 -> Mux/127
  Constant78/1 -> Mux/93
  Constant128/1 -> Mux/73
  Constant92/1 -> Mux/106
  Constant102/1 -> Mux/123
  Constant116/1 -> Mux/119
  Constant101/1 -> Mux/122
  Constant113/1 -> Mux/117
  Constant94/1 -> Mux/108
  Constant108/1 -> Mux/128
  Constant70/1 -> Mux/78
  Constant90/1 -> Mux/89
  Constant125/1 -> Mux/105
  Constant86/1 -> Mux/86
  Constant99/1 -> Mux/112
  Constant112/1 -> Mux/116
  Constant93/1 -> Mux/107
  Constant117/1 -> Mux/120
  Constant105/1 -> Mux/125
  Constant106/1 -> Mux/126
  Constant110/1 -> Mux/114
  Constant66/1 -> Mux/74
  Constant103/1 -> Mux/98
  Constant122/1 -> Mux/102
  Constant115/1 -> Mux/99
  Constant124/1 -> Mux/104
  Constant100/1 -> Mux/113
  Constant83/1 -> Mux/83
  Constant79/1 -> Mux/94
  Constant111/1 -> Mux/115
  Constant97/1 -> Mux/111
  Constant87/1 -> Mux/67
  Constant121/1 -> Mux/101
  Constant75/1 -> Mux/91
  Constant127/1 -> Mux/72
  Constant95/1 -> Mux/109
  Constant76/1 -> Mux/66
  Constant96/1 -> Mux/110
  Constant104/1 -> Mux/124
  Constant91/1 -> Mux/97
  Constant114/1 -> Mux/118
  Constant118/1 -> Mux/121
  Mux/1 -> Out1/1
